simulink model "simulink_controlador"  (R2021a)
settings: Solver=VariableStepAuto  StartTime=0.0  StopTime=9.9  RelTol=1e-3
libraries: cstblocks x3
settings Model: Creator=Pedro  LastModifiedBy=balta

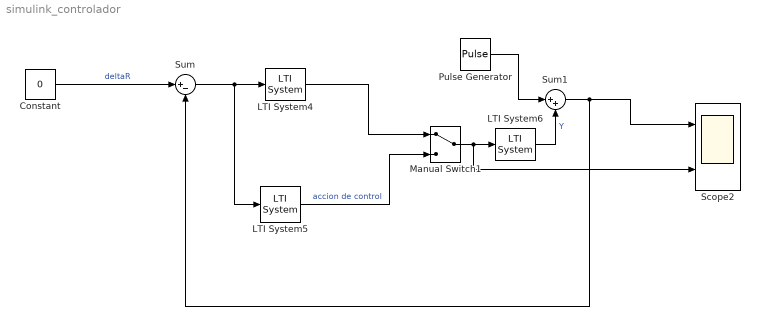
== system simulink_controlador ==
  Constant : Constant  Value=0
  LTI System4 : cstblocks/LTI System  sys=C_prop  IC=[]
  LTI System5 : cstblocks/LTI System  sys=C_PI  IC=[]
  LTI System6 : cstblocks/LTI System  sys=P  IC=[]
  Manual Switch1 : ManualSwitch
  Pulse Generator : DiscretePulseGenerator  PulseType=Time based  Amplitude=10  Period=10
  Scope2 : Scope  NumInputPorts=2
  Sum : Sum  Inputs=|+-
  Sum1 : Sum  Inputs=|++
  wires:
  LTI System6/1 -> Sum1/2  "Y"
  Sum/1 -> LTI System5/1, LTI System4/1
  Manual Switch1/1 -> Scope2/2, LTI System6/1
  LTI System5/1 -> Manual Switch1/2  "accion de control"
  Constant/1 -> Sum/1  "deltaR"
  LTI System4/1 -> Manual Switch1/1
  Pulse Generator/1 -> Sum1/1
  Sum1/1 -> Scope2/1, Sum/2
